simulink model "HIL"  (R2023b)
settings: Solver=VariableStepAuto  StartTime=0.0  StopTime=20.0  RelTol=1e-3
model workspace (MAT data in the model file):
  Iq_ref = Simulink.Parameter
  Iq_ref.Value = 0.383453146834
  Iq_ref.DataType = 'auto'
  Iq_ref.DocUnits = 'A'
  Iq_ref.Complexity = 'real'
  Iq_ref.Dimensions = [1 1]
  Ki_d = Simulink.Parameter
  Ki_d.Value = 0.000681866609844
  Ki_d.DataType = 'auto'
  Ki_d.Complexity = 'real'
  Ki_d.Dimensions = [1 1]
  Ki_q = Simulink.Parameter
  Ki_q.Value = 0
  Ki_q.DataType = 'auto'
  Ki_q.Complexity = 'real'
  Ki_q.Dimensions = [1 1]
  Kp_d = Simulink.Parameter
  Kp_d.Value = 1.11882309942
  Kp_d.DataType = 'auto'
  Kp_d.Complexity = 'real'
  Kp_d.Dimensions = [1 1]
  Kp_q = Simulink.Parameter
  Kp_q.Value = 0
  Kp_q.DataType = 'auto'
  Kp_q.Complexity = 'real'
  Kp_q.Dimensions = [1 1]
  P = Simulink.Parameter
  P.Value = 7
  P.DataType = 'auto'
  P.Complexity = 'real'
  P.Dimensions = [1 1]
  Torq = Simulink.Parameter
  Torq.Value = -0.301496617572
  Torq.DataType = 'auto'
  Torq.Complexity = 'real'
  Torq.Dimensions = [1 1]
  Vdc = Simulink.Parameter
  Vdc.Value = 24
  Vdc.DataType = 'auto'
  Vdc.DocUnits = 'V'
  Vdc.Complexity = 'real'
  Vdc.Dimensions = [1 1]
  fe = Simulink.Parameter
  fe.Value = 60
  fe.DataType = 'auto'
  fe.DocUnits = 'Hz'
  fe.Complexity = 'real'
  fe.Dimensions = [1 1]
libraries: instrumentseriallib x3, etargetslib x2, slpidlib x2, mcbcontrolslib x1, dspfdesign x1, dspstat3 x1
(part 1 of 2)
settings DebuggingCC: ParameterPrecisionLossMsg=none

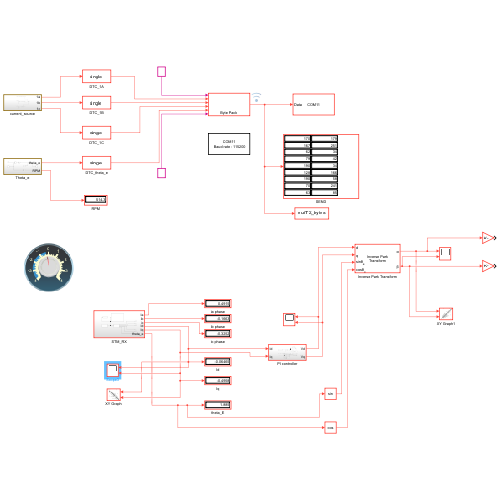
[thumbnail: Simulink's stored preview of the top-level diagram]
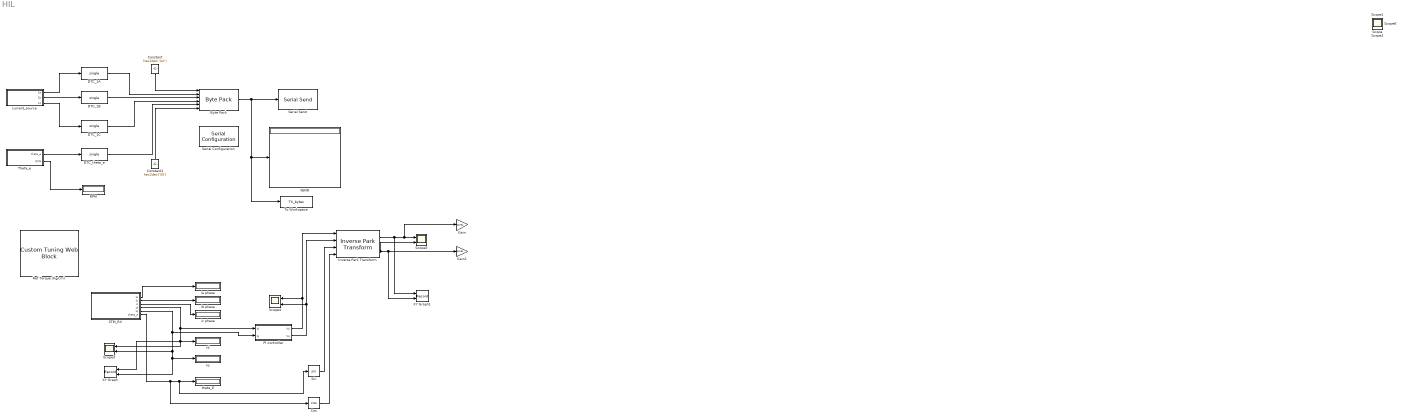
== system HIL ==
  Byte Pack : etargetslib/Byte Pack  datatypes={'uint8','single','single','single','single','uint8'}  byteAlign=1
  Constant : Constant  Value=hex2dec('AA')  OutDataTypeStr=uint8
  Constant1 : Constant  Value=hex2dec('55')  OutDataTypeStr=uint8
  Cos : Trigonometry  Operator=cos
  DTC_1A : DataTypeConversion  OutDataTypeStr=single  SaturateOnIntegerOverflow=off  RndMeth=Floor  LockScale=on
  DTC_1B : DataTypeConversion  OutDataTypeStr=single  SaturateOnIntegerOverflow=off  RndMeth=Floor  LockScale=on
  DTC_1C : DataTypeConversion  OutDataTypeStr=single  SaturateOnIntegerOverflow=off  RndMeth=Floor  LockScale=on
  DTC_theta_e : DataTypeConversion  OutDataTypeStr=single  SaturateOnIntegerOverflow=off  RndMeth=Floor  LockScale=on
  Gain : Gain  Gain=2/Vdc
  Gain1 : Gain  Gain=2/Vdc
  Id : Display
  Inverse Park Transform : mcbcontrolslib/Inverse Park Transform  PhaseInput=Two inputs  AxisAlignment=D-axis  ThetaInput=Sine and Cosine electrical position  AngleInput=Per-unit  N_points=1024
      settings: LibrarySourceBlock=mcblib/Controls/Math Transforms/Inverse Park Transform
  Iq : Display
  PI controller : Subsystem
  RPM : Display
  Ref Torque (Kg/cm) : CustomTuningWebBlock  LabelPosition=Hide  ShowInitialText=on  Configuration="{\"components\":[{\"name\":\"CircularScaleComponent\",\"settings\":{\"bounds\":{\"max\":4,\"min\":-4,\"tickInterval\":\"auto\"},\"direction\":\"cw\",\"flipLimits\":0,\"innerRadius\":0.6636618227670849,\"internalTickHeightScaleFactor\":1,\"labelColor\":[255,255,200],\"labelFont\":{\"font\":\"Arial\",\"fontSize\":12},\"labelRadius\":0.7741084267289068,\"labelTransparency\":1,\"minorTickHeightScaleFactor\":0.2,\"needleImage\":{\"size\":[150,150],\"src\":\"data:image\\/svg+xml;base64,PD94bWwgdmVyc2lvbj0iMS4wIiBlbmNvZGluZz0idXRmLTgiPz4NCjwhLS0gR2VuZXJhdG9yOiBBZG9iZSBJbGx1c3RyYXRvciAyNS4yLjMsIFNWRyBFeHBvcnQgUGx1Zy1JbiAuIFNWRyBWZXJzaW9uOiA2LjAwIEJ1aWxkIDApICAtLT4NCjxzdmcgdmVyc2lvbj0iMS4xIiBpZD0iTGF5ZXJfMSIgeG1sbnM9Imh0dHA6Ly93d3cudzMub3JnLzIwMDAvc3ZnIiB4bWxuczp4bGluaz0iaHR0cDovL3d3dy53My5vcmcvMTk5OS94bGluayIgeD0iMHB4IiB5PSIwcHgiDQoJIHZpZXdCb3g9IjAgMCAxNTIgMTUyIiBzdHlsZT0iZW5hYmxl ...(+37472 chars)\"},\"needleOffset\":[-0.008064516129032258,0],\"needleOrientation\":-45,\"needleRotation\":90,\"needleSize\":{\"height\":0.44,\"width\":0.44},\"outerRadius\":0.4782608695652174,\"position\":[0,0,1,1],\"referencePoint\":\"auto\",\"scaleAngle\":270,\"scaleAngleOffset\":135,\"scaleColors\":[],\"scaleColorsSize\":0.2,\"scaleDirection\":\"CW\",\"scalePosition\":[0,0,1,1],\"showLabels\":1,\"showMinorTicks\":1,\"showSpanLine\":true,\"showTicks\":1,\"tickColor\":[252,252,197],\"tickTransparency\":1,\"valueBarColor\":[0,114,189],\"valueBarPosition\":[0,0,1,1],\"valueBarSize\":0.2,\"valueBarTransparency\":1}},{\"name\":\"BackgroundImageComponent\",\"settings\":{\"image\":{\"size\":[385,373],\"src\":\"data:image\\/svg+xml;base64,PD94bWwgdmVyc2lvbj0iMS4wIiBlbmNvZGluZz0idXRmLTgiPz4NCjwhLS0gR2VuZXJhdG9yOiBBZG9iZSBJbGx1c3RyYXRvciAyNS4wLjAsIFNWRyBFeHBvcnQgUGx1Zy1JbiAuIFNWRyBWZXJzaW9uOiA2LjAwIEJ1aWxkIDApICAtLT4NCjxzdmcgdmVyc2lvbj0iMS4xIg0KCSBpZD0iTGF5ZXJfMl8xXyIgeG1sbnM6Y2M9Imh0dHA6Ly9jcmVhdGl2ZWNvbW1vbnMub3JnL25zIyIgeG1sbnM6ZGM9Imh0dHA6Ly9wdXJsLm9yZy9kYy9lbGVtZW50cy8xLjEvIiB4bWxuczppbmtzY2FwZT0iaHR0cDovL3d3dy5pbmtzY2FwZS5vcmcv ...(+4184 chars)\",\"srcOrientation\":\"horizontal\"},\"position\":[0,0,1,1],\"scaleMode\":\"0\"}},{\"name\":\"ForegroundImageComponent\",\"settings\":{\"image\":{\"size\":[0,0],\"src\":\"default\",\"srcOrientation\":[]},\"isForeground\":1,\"position\":[0,0,1,1],\"scaleMode\":\"0\"}}],\"settings\":{\"BindingType\":\"param\",\"aspectRatio\":1,\"backgroundColor\":[0,0,0,\"1\"],\"backgroundOffset\":1,\"backgroundOpacity\":1,\"direction\":\"cw\",\"fixedAspectRatio\":\"on\",\"flipLimits\":0,\"foregroundColor\":[252,252,196],\"orientation\":\"horizontal\",\"showBackgroundColor\":false,\"value\":0,\"version\":\"R2023a\"},\"type\":\"CircularGauge\"}"
  SEND : Display
  STM_RX : Subsystem
  Scope3 : Scope  NumInputPorts=2
  Scope4 : Scope  NumInputPorts=2
  Scope5 : Scope  NumInputPorts=2
  Serial Configuration : instrumentseriallib/Serial Configuration  Priority=-200000  PortSel=COM11  Port=COM11  ComPort=COM11  BaudRate=115200  DataBits=8  Parity=none  StopBits=1  ByteOrder=little-endian  FlowControl=none  Timeout=10  SimulateUsing=Interpreted execution  BlockInModel=on  aMode=1
      settings: LibrarySourceBlock=embeddedtargetslib/Host Communication/Serial Configuration
  Serial Send : instrumentseriallib/Serial Send  Priority=1  PortSel=COM11  Port=COM11  ComPort=COM11  Header=[]  Terminator=<none>  CustomTerminator=[]  EnableBlockingMode=on  SimulateUsing=Interpreted execution  BlockInModel=on  aMode=1
      settings: LibrarySourceBlock=embeddedtargetslib/Host Communication/Serial Send
  Sin : Trigonometry
  Theta_e : Subsystem
  To Workspace : ToWorkspace  VariableName=TX_bytes  SampleTime=-1
  XY Graph : Record  FileSettingsInternal="{\"entries\":[{\"content\":{\"excelSettings\":{\"content\":{},\"type\":\"Streamout.ExcelSettings\"}},\"type\":\"Streamout.FileSettingStorage\",\"uuid\":\"\"}],\"packageUris\":[\"http:\\/\\/schema.mathworks.com\\/mf0\\/streamout_blocks\\/R2020a\"],\"version\":\"1.0\"}"  Layout=[1 1]  SignalsInternal="{\"entries\":[{\"content\":{\"signals\":[{\"content\":{\"blockPath\":[],\"dimensions\":[1,1],\"domain\":\"\",\"lineColor\":\"#a2142f\",\"plots\":[1],\"port\":1,\"sid\":[\"\"],\"signalID\":39,\"signalName\":\"STM_RX:4\"},\"type\":\"RecordBlkView.Signal\",\"uuid\":\"\"},{\"content\":{\"blockPath\":[],\"dimensions\":[1,1],\"domain\":\"\",\"lineColor\":\"#139fff\",\"plots\":[1],\"port\":2,\"sid\":[\"\"],\"signalID\":43,\"signalName\":\"STM_RX:5\"},\"type\":\"RecordBlkView.Signal\",\"uuid\":\"\"}]},\"type\":\"RecordBlkView.InputSignals\",\"uuid\":\"\"}],\"packageUris\":[\"http:\\/\\/schema.mathworks.com\\/mf0\\/streamout_blocks\\/R2020a\"],\"version\":\"1.0\"}"  VisualizationBindings="{\"xyplotplugin\":{\"info\":[{\"series\":[{\"bindingParametersList\":[{\"parameter\":\"X-Axis\",\"signalID\":39,\"signalName\":\"STM_RX:4\"},{\"parameter\":\"Y-Axis\",\"signalID\":43,\"signalName\":\"STM_RX:5\"}],\"seriesID\":24392}],\"subplotID\":1}]}}"  CompatibilityTag=XY
  XY Graph1 : Record  FileSettingsInternal="{\"entries\":[{\"content\":{\"excelSettings\":{\"content\":{},\"type\":\"Streamout.ExcelSettings\"}},\"type\":\"Streamout.FileSettingStorage\",\"uuid\":\"\"}],\"packageUris\":[\"http:\\/\\/schema.mathworks.com\\/mf0\\/streamout_blocks\\/R2020a\"],\"version\":\"1.0\"}"  Layout=[1 1]  SignalsInternal="{\"entries\":[{\"content\":{\"signals\":[{\"content\":{\"blockPath\":[],\"dimensions\":[1],\"domain\":\"\",\"lineColor\":\"#a2142f\",\"plots\":[1],\"port\":1,\"sid\":[\"\"],\"signalID\":47,\"signalName\":\"Inverse Park Transform:1\"},\"type\":\"RecordBlkView.Signal\",\"uuid\":\"\"},{\"content\":{\"blockPath\":[],\"dimensions\":[1],\"domain\":\"\",\"lineColor\":\"#139fff\",\"plots\":[1],\"port\":2,\"sid\":[\"\"],\"signalID\":51,\"signalName\":\"Inverse Park Transform:2\"},\"type\":\"RecordBlkView.Signal\",\"uuid\":\"\"}]},\"type\":\"RecordBlkView.InputSignals\",\"uuid\":\"\"}],\"packageUris\":[\"http:\\/\\/schema.mathworks.com\\/mf0\\/streamout_blocks\\/R2020a\"],\"version\":\"1.0\"}"  VisualizationBindings="{\"xyplotplugin\":{\"info\":[{\"series\":[{\"bindingParametersList\":[{\"parameter\":\"X-Axis\",\"signalID\":47,\"signalName\":\"Inverse Park Transform:1\"},{\"parameter\":\"Y-Axis\",\"signalID\":51,\"signalName\":\"Inverse Park Transform:2\"}],\"seriesID\":62696}],\"subplotID\":1}]}}"  CompatibilityTag=XY
  current_source : Subsystem
  ia phase : Display
  ib phase : Display
  ic phase : Display
  theta_E : Display
  Scope{,1..2,6} (4 alike) : Scope
  wires:
  current_source/1(1a) -> DTC_1A/1
  current_source/2(1b) -> DTC_1B/1
  current_source/3(1c) -> DTC_1C/1
  Byte Pack/1 -> To Workspace/1, SEND/1, Serial Send/1
  Constant/1 -> Byte Pack/1
  DTC_1B/1 -> Byte Pack/3
  DTC_1A/1 -> Byte Pack/2
  DTC_1C/1 -> Byte Pack/4
  Theta_e/1(theta_e) -> DTC_theta_e/1
  Theta_e/2(RPM) -> RPM/1
  Constant1/1 -> Byte Pack/6
  DTC_theta_e/1 -> Byte Pack/5
  STM_RX/4(Id) -> XY Graph/1, Scope3/1, Id/1, PI controller/1(Id)
  STM_RX/5(Iq) -> Iq/1, XY Graph/2, Scope3/2, PI controller/2(Iq)
  STM_RX/3(ic) -> ic phase/1
  STM_RX/2(ib) -> ib phase/1
  STM_RX/1(Ia) -> ia phase/1
  STM_RX/6(theta_e) -> Cos/1, theta_E/1, Sin/1
  PI controller/1(Vd) -> Scope4/1, Inverse Park Transform/1
  PI controller/2(Vq) -> Inverse Park Transform/2, Scope4/2
  Cos/1 -> Inverse Park Transform/4
  Sin/1 -> Inverse Park Transform/3
  Inverse Park Transform/1 -> XY Graph1/1, Gain/1, Scope5/1
  Inverse Park Transform/2 -> Scope5/2, Gain1/1, XY Graph1/2
